simulink model "untitled"  (R2025b)
settings: Solver=VariableStepAuto  StartTime=0.0  StopTime=10  RelTol=1e-3

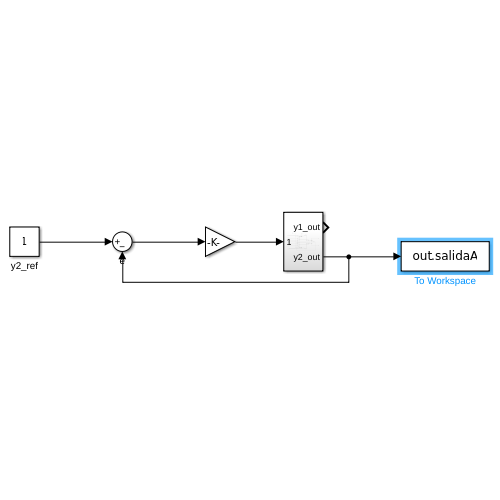
[thumbnail: Simulink's stored preview of the top-level diagram]
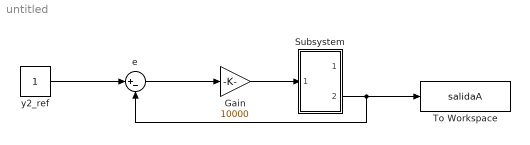
== system untitled ==
  Gain : Gain  Gain=10000
  Subsystem : Subsystem
  To Workspace : ToWorkspace  VariableName=salidaA  SaveFormat=Structure With Time  SampleTime=-1
  e : Sum  Inputs=|+-
  y2_ref : Constant
  wires:
  e/1 -> Gain/1
  y2_ref/1 -> e/1
  Gain/1 -> Subsystem/1(In1)
  Subsystem/2(y2_out) -> e/2, To Workspace/1

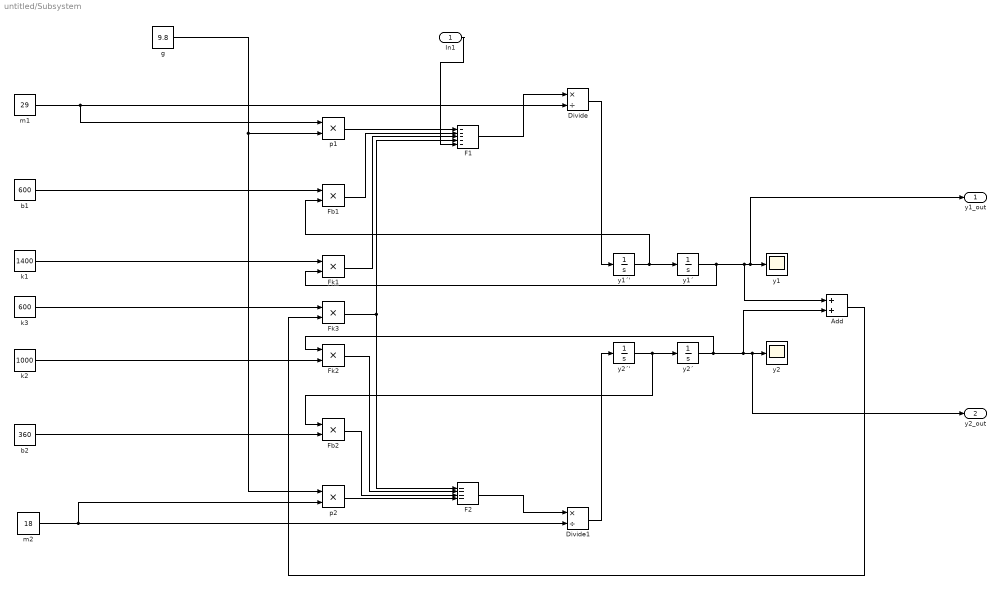
== system untitled/Subsystem ==
  In1 : Inport
  Add : Sum
  Divide : Product  Inputs=*/
  Divide1 : Product  Inputs=*/
  F1 : Sum  Inputs=-----
  F2 : Sum  Inputs=----
  Fb1 : Product
  Fb2 : Product
  Fk1 : Product
  Fk2 : Product
  Fk3 : Product
  b1 : Constant  Value=600
  b2 : Constant  Value=360
  g : Constant  Value=9.8
  k1 : Constant  Value=1400
  k2 : Constant  Value=1000
  k3 : Constant  Value=600
  m1 : Constant  Value=29
  m2 : Constant  Value=18
  p1 : Product
  p2 : Product
  y1 : Scope
      settings: ActiveDisplayYMinimum=-0.13821241316017782  ActiveDisplayYMaximum=0.01535693479557531
  y1´ : Integrator
  y1´' : Integrator
  y2 : Scope
      settings: ActiveDisplayYMinimum=-0.085497340731502447  ActiveDisplayYMaximum=0.0094997045257224928
  y2´ : Integrator
  y2´' : Integrator
  y1_out : Outport
  y2_out : Outport  Port=2
  wires:
  Divide1/1 -> y2´'/1
  b2/1 -> Fb2/2
  p1/1 -> F1/1
  k2/1 -> Fk2/2
  b1/1 -> Fb1/1
  In1/1 -> F1/5
  y1´'/1 -> Fb1/2, y1´/1
  Fb1/1 -> F1/2
  Fk3/1 -> F1/4, F2/1
  k1/1 -> Fk1/1
  y1´/1 -> Fk1/2, Add/1, y1_out/1, y1/1
  Fb2/1 -> F2/3
  m2/1 -> p2/2, Divide1/2
  y2´'/1 -> Fb2/1, y2´/1
  F2/1 -> Divide1/1
  y2´/1 -> Fk2/1, Add/2, y2_out/1, y2/1
  k3/1 -> Fk3/1
  Fk1/1 -> F1/3
  p2/1 -> F2/4
  m1/1 -> p1/1, Divide/2
  F1/1 -> Divide/1
  Add/1 -> Fk3/2
  Fk2/1 -> F2/2
  Divide/1 -> y1´'/1
  g/1 -> p1/2, p2/1
